simulink model "phxex_sim_ballplate2"  (R2026a)
settings: Solver=FixedStepDiscrete  StopTime=36  FixedStep=0.005
values from neighbouring files (symbols this model uses):
  Bowl = phx.Body("Type", "kinematic", "Position", [0 0 0],          "Shape", {"Revolution", "Profile", prof, "Axis", "z", "Envelope", "concave", "Color", [0.82 0.85 0.90], "Texture", "checker", "TextureBlend", 0.5},          "Friction", [0.6 0 0], "Name", "Bowl")    [model_ballplate2.m]
libraries: PhxLibrary x1
settings Model: Creator=lzhan  LastModifiedBy=lzhan

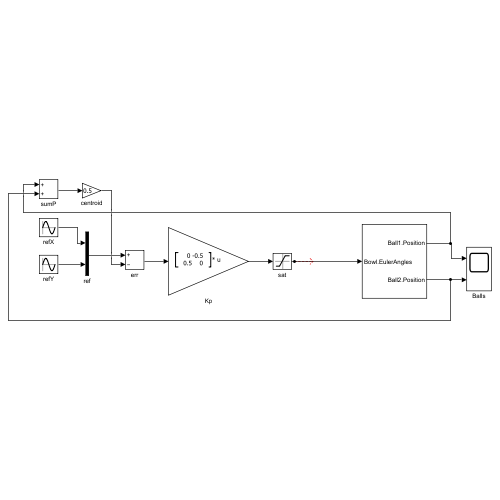
[thumbnail: Simulink's stored preview of the top-level diagram]
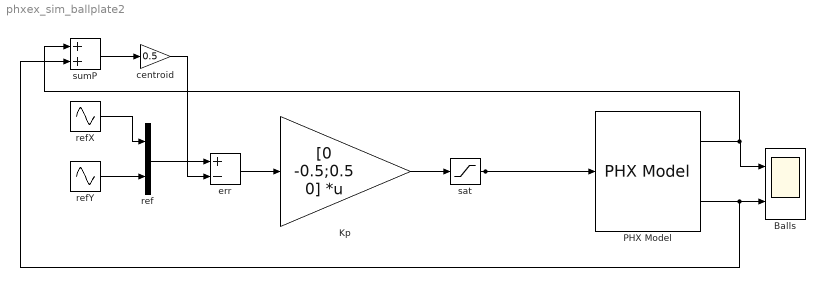
== system phxex_sim_ballplate2 ==
  Balls : Scope  NumInputPorts=2
      settings: ActiveDisplayYMinimum=-1  ActiveDisplayYMaximum=1
  Kp : Gain  Gain=[0 -0.5;0.5 0]  Multiplication=Matrix(K*u)
  PHX Model : PhxLibrary/PHX Model  ModelSource=saved_ballplate2.mat  InputRefs=Bowl.EulerAngles(1:2)  OutputRefs=|  ShowViewer=on  RenderEach=on  CameraPosition=[-15,-15,15]  CameraTarget=[0,0,2]  SimulationStep=0.01  SimpleIcon=off  Substeps=1  CameraResolution=[0 0]
      | Ball1.Position(1:2)
      | Ball2.Position(1:2)
      settings: SourceProductName=PHX Toolbox
  centroid : Gain  Gain=0.5
  err : Sum  Inputs=+-
  ref : Mux  Inputs=2
  refX : Sin  Amplitude=3  Frequency=0.34907  SampleTime=0
  refY : Sin  Amplitude=1.5  Bias=1.5  Frequency=0.34907  Phase=-1.5708  SampleTime=0
  sat : Saturate  UpperLimit=0.25  LowerLimit=-0.25
  sumP : Sum
  wires:
  sumP/1 -> centroid/1
  sat/1 -> PHX Model/1
  ref/1 -> err/1
  refY/1 -> ref/2
  PHX Model/1 -> Balls/1, sumP/1
  centroid/1 -> err/2
  err/1 -> Kp/1
  refX/1 -> ref/1
  Kp/1 -> sat/1
  PHX Model/2 -> sumP/2, Balls/2
